simulink model "SimulationExampleWithFIU"  (Simulink 8.0)
settings: Solver=FixedStepDiscrete  SolverMode=SingleTasking  StartTime=0.0  StopTime=10  FixedStep=0.001  RelTol=1e-3
libraries: FaultInsertionUnit x1, simulink x1
settings Model: Creator=jroth  LastModifiedBy=jroth

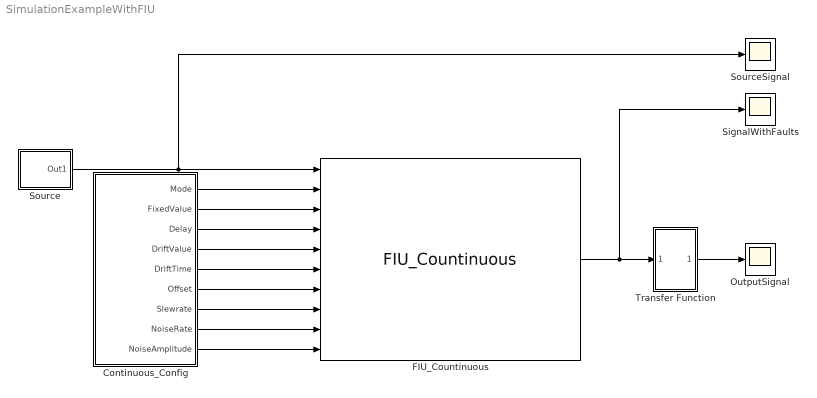
== system SimulationExampleWithFIU ==
  Continuous_Config : Subsystem
  FIU_Countinuous : FaultInsertionUnit/FIU_Countinuous
  OutputSignal : Scope
      settings: MaxDataPoints=50000
  SignalWithFaults : Scope
      settings: SaveName=ScopeData2  MaxDataPoints=50000
  Source : Subsystem
  SourceSignal : Scope
      settings: MaxDataPoints=50000
  Transfer Function : Subsystem
  wires:
  Transfer Function/1(Out1) -> OutputSignal/1
  Source/1(Out1) -> SourceSignal/1, FIU_Countinuous/1
  FIU_Countinuous/1 -> SignalWithFaults/1, Transfer Function/1(In1)
  Continuous_Config/9(NoiseAmplitude) -> FIU_Countinuous/10
  Continuous_Config/8(NoiseRate) -> FIU_Countinuous/9
  Continuous_Config/7(Slewrate) -> FIU_Countinuous/8
  Continuous_Config/6(Offset) -> FIU_Countinuous/7
  Continuous_Config/5(DriftTime) -> FIU_Countinuous/6
  Continuous_Config/4(DriftValue) -> FIU_Countinuous/5
  Continuous_Config/3(Delay) -> FIU_Countinuous/4
  Continuous_Config/2(FixedValue) -> FIU_Countinuous/3
  Continuous_Config/1(Mode) -> FIU_Countinuous/2

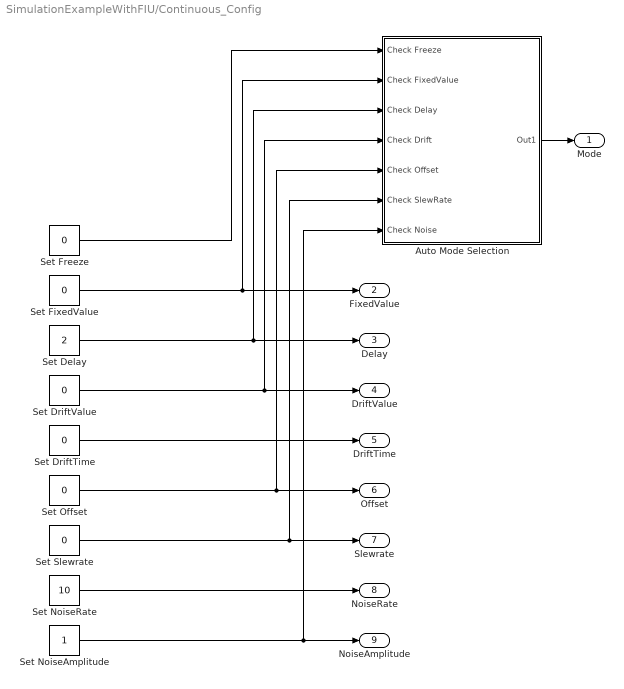
== system SimulationExampleWithFIU/Continuous_Config ==
  Auto Mode Selection : Subsystem
  Set Delay : Constant  Value=2
  Set DriftTime : Constant  Value=0
  Set DriftValue : Constant  Value=0
  Set FixedValue : Constant  Value=0
  Set Freeze : Constant  Value=0
  Set NoiseAmplitude : Constant
  Set NoiseRate : Constant  Value=10
  Set Offset : Constant  Value=0
  Set Slewrate : Constant  Value=0
  Mode : Outport
  FixedValue : Outport  Port=2
  Delay : Outport  Port=3
  DriftValue : Outport  Port=4
  DriftTime : Outport  Port=5
  Offset : Outport  Port=6
  Slewrate : Outport  Port=7
  NoiseRate : Outport  Port=8
  NoiseAmplitude : Outport  Port=9
  wires:
  Set NoiseRate/1 -> NoiseRate/1
  Set Delay/1 -> Auto Mode Selection/3(Check Delay), Delay/1
  Set Offset/1 -> Auto Mode Selection/5(Check Offset), Offset/1
  Set FixedValue/1 -> Auto Mode Selection/2(Check FixedValue), FixedValue/1
  Set NoiseAmplitude/1 -> Auto Mode Selection/7(Check Noise), NoiseAmplitude/1
  Set Slewrate/1 -> Auto Mode Selection/6(Check SlewRate), Slewrate/1
  Auto Mode Selection/1(Out1) -> Mode/1
  Set DriftValue/1 -> Auto Mode Selection/4(Check Drift), DriftValue/1
  Set DriftTime/1 -> DriftTime/1
  Set Freeze/1 -> Auto Mode Selection/1(Check Freeze)

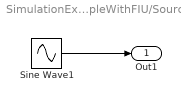
== system SimulationExampleWithFIU/Source ==
  Sine Wave1 : Sin  Amplitude=2  Frequency=2  SampleTime=0
  Out1 : Outport
  wires:
  Sine Wave1/1 -> Out1/1

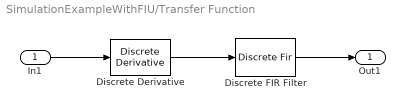
== system SimulationExampleWithFIU/Transfer Function ==
  In1 : Inport
  Discrete Derivative : simulink/Discrete/Discrete Derivative  gainval=1.0  ICPrevScaledInput=0.0  InputProcessing=Inherited  OutMin=[]  OutMax=[]  OutDataType=fixdt(1, 16)  OutScaling=2^-10  DoSatur=off
  Discrete FIR Filter : DiscreteFir  Coefficients=[1 0.2]
  Out1 : Outport
  wires:
  In1/1 -> Discrete Derivative/1
  Discrete Derivative/1 -> Discrete FIR Filter/1
  Discrete FIR Filter/1 -> Out1/1

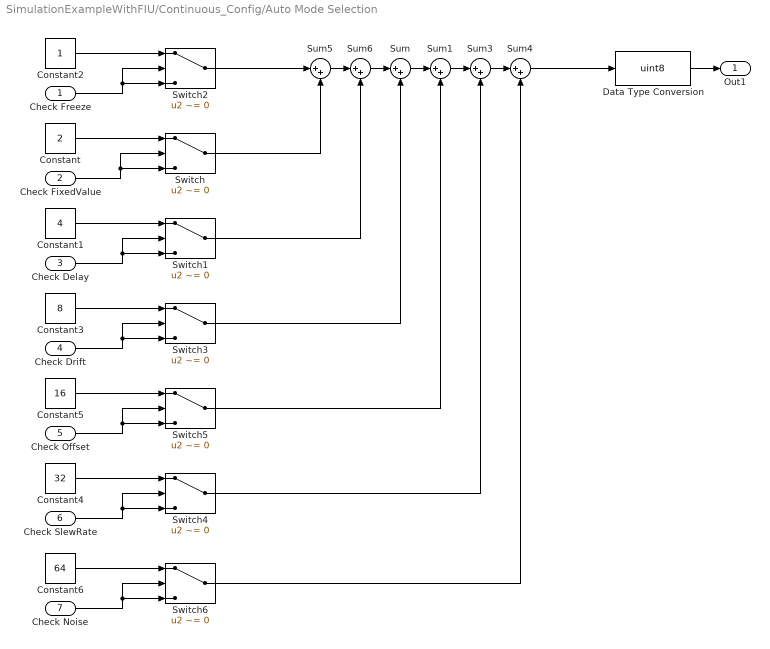
== system SimulationExampleWithFIU/Continuous_Config/Auto Mode Selection ==
  Check Freeze : Inport
  Check FixedValue : Inport  Port=2
  Check Delay : Inport  Port=3
  Check Drift : Inport  Port=4
  Check Offset : Inport  Port=5
  Check SlewRate : Inport  Port=6
  Check Noise : Inport  Port=7
  Constant : Constant  Value=2
  Constant1 : Constant  Value=4
  Constant2 : Constant
  Constant3 : Constant  Value=8
  Constant4 : Constant  Value=32
  Constant5 : Constant  Value=16
  Constant6 : Constant  Value=64
  Data Type Conversion : DataTypeConversion  OutDataTypeStr=uint8
  Sum{,1,3..6} (6 alike) : Sum  Inputs=|++
  Switch{,1..6} (7 alike) : Switch  Criteria=u2 ~= 0
  Out1 : Outport
  wires:
  Sum1/1 -> Sum3/1
  Constant2/1 -> Switch2/1
  Sum3/1 -> Sum4/1
  Sum/1 -> Sum1/1
  Check Drift/1 -> Switch3/3, Switch3/2
  Check Freeze/1 -> Switch2/3, Switch2/2
  Check Delay/1 -> Switch1/3, Switch1/2
  Check SlewRate/1 -> Switch4/3, Switch4/2
  Check FixedValue/1 -> Switch/3, Switch/2
  Constant/1 -> Switch/1
  Constant4/1 -> Switch4/1
  Constant1/1 -> Switch1/1
  Constant3/1 -> Switch3/1
  Data Type Conversion/1 -> Out1/1
  Check Offset/1 -> Switch5/3, Switch5/2
  Constant5/1 -> Switch5/1
  Sum4/1 -> Data Type Conversion/1
  Check Noise/1 -> Switch6/3, Switch6/2
  Constant6/1 -> Switch6/1
  Sum5/1 -> Sum6/1
  Sum6/1 -> Sum/1
  Switch2/1 -> Sum5/1
  Switch/1 -> Sum5/2
  Switch1/1 -> Sum6/2
  Switch3/1 -> Sum/2
  Switch5/1 -> Sum1/2
  Switch4/1 -> Sum3/2
  Switch6/1 -> Sum4/2
